simulink model "Esys"  (R2015a)
settings: Solver=ode45  StartTime=0.0  StopTime=5  RelTol=1e-6  AbsTol=1e-6
values from neighbouring files (symbols this model uses):
  C1_ref = block.DialogPrm(6).Data    [Esys_S_m.m]    (also in Parameter.m = 1e-06)
  C2 = block.DialogPrm(9).Data    [Esys_S_m.m]    (also in Parameter.m = 1e-06)
  K = block.DialogPrm(5).Data    [Esys_S_m.m]    (also in Parameter.m = 3)
  kC1 = block.DialogPrm(8).Data    [Esys_S_m.m]    (also in Parameter.m = 8e-07)
  R1 = block.DialogPrm(3).Data    [Esys_S_m.m]    (also in Parameter.m = 625)
  R2 = block.DialogPrm(4).Data    [Esys_S_m.m]    (also in Parameter.m = 3500)
  te = 1    [Parameter.m]
  ts = 3    [Parameter.m]
  UC1_ref = block.DialogPrm(7).Data    [Esys_S_m.m]    (also in Parameter.m = -10)
  Ue = u(1)    [Esys_S_m.m]    (also in Parameter.m = 7)
  UeR = 5    [Parameter.m]
  Us = u(2)    [Esys_S_m.m]    (also in Parameter.m = 1)
  Usinus = 0.1    [Parameter.m]
  UsR = 5    [Parameter.m]
  we = 10    [Parameter.m]
undefined symbols (not defined in the file or in its folder): UC1R, UC2R
settings Model: Creator=sj  LastModifiedBy=sj

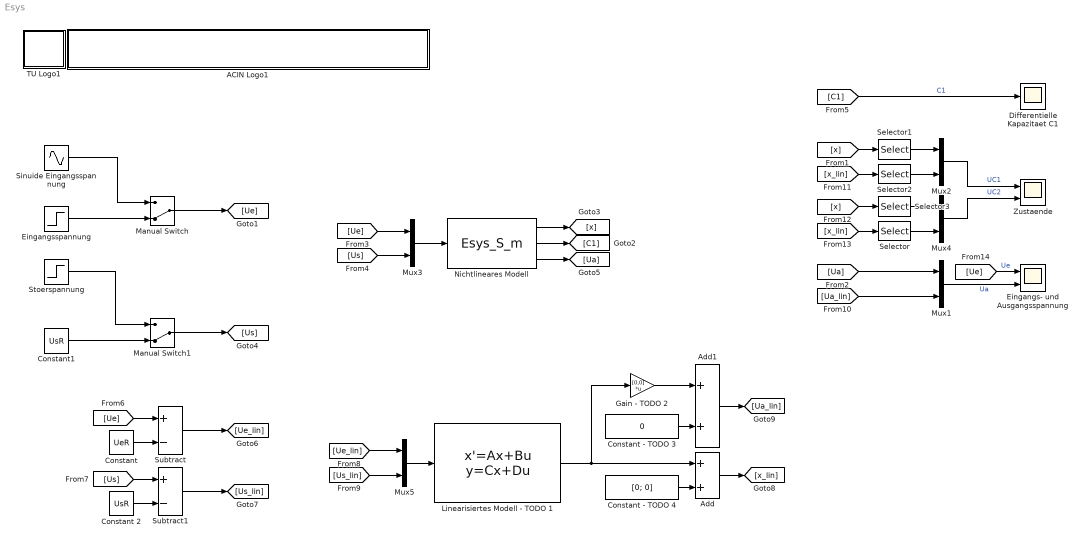
== system Esys ==
  ACIN Logo1 : Subsystem
      mask init:
      | s = get_param(gcb,'UserData');
      mask Display:
      | image(s.logo,[0 0 439 45]);
      | %axis image
  Add : Sum
  Add1 : Sum
  Constant : Constant  Value=UeR
  Constant - TODO 3 : Constant  Value=0
  Constant - TODO 4 : Constant  Value=[0; 0]
  Constant 2 : Constant  Value=UsR
  Constant1 : Constant  Value=UsR
  Differentielle Kapazitaet C1 : Scope
      settings: TimeRange=20  YMin=2.5e-06  YMax=4.1e-06  SaveName=ScopeData3
  Eingangs- und Ausgangsspannung : Scope  NumInputPorts=2
      settings: TimeRange=20  YMin=4.9~14.9  YMax=5.100000000000001~15.1
  Eingangsspannung : Step  Time=te  Before=UeR  After=Ue  SampleTime=0
  Gain - TODO 2 : Gain  Gain=[0,0]  Multiplication=Matrix(K*u)
  Linearisiertes Modell - TODO 1 : StateSpace  A=zeros(2)  B=zeros(2)  C=zeros(2)  D=zeros(2)  X0=[0;0]
  Manual Switch : ManualSwitch  CurrentSetting=0
  Manual Switch1 : ManualSwitch  CurrentSetting=0
  Mux{1..5} (5 alike) : Mux  Inputs=2
  Nichtlineares Modell : M-S-Function  FunctionName=Esys_S_m  Parameters=UC1R,UC2R,R1,R2,K,C1_ref,UC1_ref,kC1,C2  mask{UC10=UC1R, UC20=UC2R, R1=R1, R2=R2, K=K, C1_ref=C1_ref, UC1_ref=UC1_ref, kC1=kC1, C2=C2}
      mask prompts: UC10 "Anfangswert von UC1 in Volt"; UC20 "Anfangswert von UC2 in Volt"; R1 "Widerstand R1 in Ohm"; R2 "Widerstand R2 in Ohm"; K "Spannungsverstärkung K"; C1_ref "Kapazitäts-Referenzwert auf Kennlinie von C1 in F"; UC1_ref "Spannungs-Referenzwert auf Kennlinie von C1 in V"; kC1 "Steigung der Kennlinie in F/V"; C2 "Kapazität C2 in F"
      mask DialogControl Container3 Prompt: Nichtlineare Kapazität C1
  Selector : Selector  InputPortWidth=2  Indices=2
  Selector1 : Selector  InputPortWidth=2
  Selector2 : Selector  InputPortWidth=2
  Selector3 : Selector  InputPortWidth=2  Indices=2
  Sinuide Eingangsspannung : Sin  Amplitude=Usinus  Bias=UeR  Frequency=we  SampleTime=0
  Stoerspannung : Step  Time=ts  Before=UsR  After=Us  SampleTime=0
  Subtract : Sum  Inputs=+-
  Subtract1 : Sum  Inputs=+-
  TU Logo1 : Subsystem
      mask init:
      | s = get_param(gcb,'UserData');
      mask Display: image(s.logo,[0 0 45 45]);
  Zustaende : Scope  NumInputPorts=2
      settings: TimeRange=20  YMin=-12.5~4  YMax=-3.5~7.5  SaveName=ScopeData2
  wires:
  Mux3/1 -> Nichtlineares Modell/1
  Nichtlineares Modell/1 -> [x]
  Nichtlineares Modell/2 -> [C1]
  [Ue] -> Mux3/1
  [Us] -> Mux3/2
  Eingangsspannung/1 -> Manual Switch/2
  Sinuide Eingangsspannung/1 -> Manual Switch/1
  Manual Switch/1 -> [Ue]
  Nichtlineares Modell/3 -> [Ua]
  [C1] -> Differentielle Kapazitaet C1/1  "C1"
  Subtract/1 -> [Ue_lin]
  Constant/1 -> Subtract/2
  [Ue] -> Subtract/1
  Subtract1/1 -> [Us_lin]
  Constant 2/1 -> Subtract1/2
  [Us] -> Subtract1/1
  Linearisiertes Modell - TODO 1/1 -> Gain - TODO 2/1, Add/1
  Mux5/1 -> Linearisiertes Modell - TODO 1/1
  [Ue_lin] -> Mux5/1
  [Us_lin] -> Mux5/2
  Add/1 -> [x_lin]
  Constant - TODO 4/1 -> Add/2
  Gain - TODO 2/1 -> Add1/1
  Constant - TODO 3/1 -> Add1/2
  Add1/1 -> [Ua_lin]
  [Ua] -> Mux1/1
  [Ua_lin] -> Mux1/2
  Selector1/1 -> Mux2/1
  Selector2/1 -> Mux2/2
  [x] -> Selector1/1
  [x_lin] -> Selector2/1
  Selector3/1 -> Mux4/1
  Selector/1 -> Mux4/2
  [x] -> Selector3/1
  [x_lin] -> Selector/1
  Mux2/1 -> Zustaende/1  "UC1"
  Mux4/1 -> Zustaende/2  "UC2"
  [Ue] -> Eingangs- und Ausgangsspannung/1  "Ue"
  Mux1/1 -> Eingangs- und Ausgangsspannung/2  "Ua"
  Manual Switch1/1 -> [Us]
  Stoerspannung/1 -> Manual Switch1/1
  Constant1/1 -> Manual Switch1/2

== system Esys/ACIN Logo1 ==

== system Esys/TU Logo1 ==
